simulink model "sampleModel1766"  (R2023a)
settings: Solver=VariableStepAuto  StartTime=0.0  StopTime=10.0  RelTol=1e-3
libraries: hdlsllib x6, simulink x2
settings Model: Creator=user1  LastModifiedBy=user1

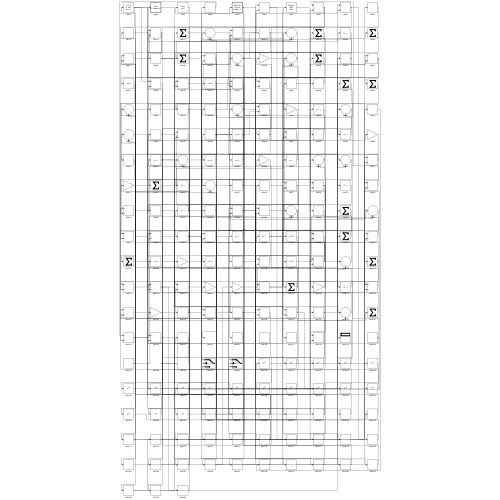
[thumbnail: Simulink's stored preview of the top-level diagram]
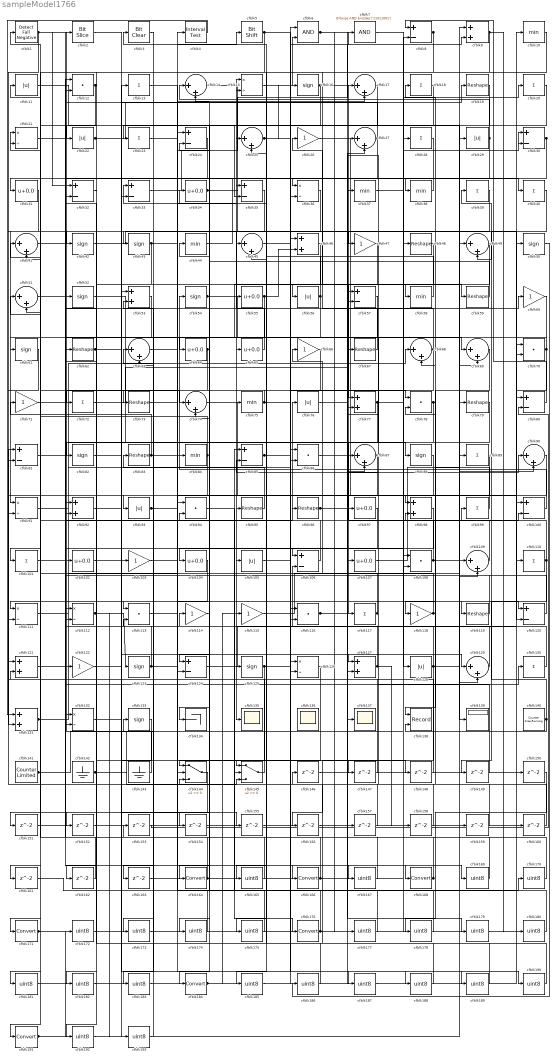
== system sampleModel1766 ==
  cfblk1 : hdlsllib/Logic and Bit Operations/Detect Fall Negative  vinit=0  OutDataTypeStr=boolean
  cfblk{10,37..38,44,58,75,84} (7 alike) : MinMax
  cfblk{8,24,30,32..33,35,57,80..81,85,100,106,120,124} (14 alike) : Sum  Inputs=+-
  cfblk{13,18,20,23,28,39..40,72,89,99,101,110,117,130} (14 alike) : Sum  Inputs=+
  cfblk{31,34,55,64..65,97,102,104,107} (9 alike) : Bias  Bias=0.0  SaturateOnIntegerOverflow=off
  cfblk{26,47,60,66,71,103,114..115,118,122} (10 alike) : Gain
  cfblk{11,22,29,56,76,93,105,128} (8 alike) : Abs  SaturateOnIntegerOverflow=off
  cfblk{12,70,78,86,94,108,113,116} (8 alike) : DotProduct  OutDataTypeStr=Inherit: Inherit via internal rule
  cfblk{14,17,25,27,41,45,49,51,63,68..69,74,87,90,109,129} (16 alike) : Sum  Inputs=|++
  cfblk{15,21,36,91,111..112,126,132} (8 alike) : Product  Inputs=*/  RndMeth=Zero  SaturateOnIntegerOverflow=on
  cfblk{19,48,59,62,67,73,79,83,95..96,119} (11 alike) : Reshape
  cfblk{9,46,53,77,92,98,121,127,131} (9 alike) : Sum
  cfblk{16,42..43,50,52,54,61,82,88,123,125,133} (12 alike) : Signum
  cfblk134 : Terminator
  cfblk135 : Scope
  cfblk136 : Scope
      settings: Floating=on
  cfblk137 : Scope
  cfblk138 : Record  FileSettingsInternal="{\"entries\":[{\"content\":{\"excelSettings\":{\"content\":{},\"type\":\"Streamout.ExcelSettings\"}},\"type\":\"Streamout.FileSettingStorage\",\"uuid\":\"\"}],\"packageUris\":[\"http:\\/\\/schema.mathworks.com\\/mf0\\/streamout_blocks\\/R2020a\"],\"version\":\"1.0\"}"  Layout=[1 1]  SignalsInternal="{\"entries\":[{\"content\":{\"signals\":[{\"content\":{\"blockPath\":[],\"dimensions\":[1],\"domain\":\"\",\"lineColor\":\"#a2142f\",\"plots\":[1],\"port\":1,\"signalID\":3847,\"signalName\":\"XY Graph:1\"},\"type\":\"RecordBlkView.Signal\",\"uuid\":\"\"},{\"content\":{\"blockPath\":[],\"dimensions\":[1],\"domain\":\"\",\"lineColor\":\"#139fff\",\"plots\":[1],\"port\":2,\"signalID\":3850,\"signalName\":\"XY Graph:2\"},\"type\":\"RecordBlkView.Signal\",\"uuid\":\"\"}]},\"type\":\"RecordBlkView.InputSignals\",\"uuid\":\"\"}],\"packageUris\":[\"http:\\/\\/schema.mathworks.com\\/mf0\\/streamout_blocks\\/R2020a\"],\"version\":\"1.0\"}"  VisualizationBindings="{\"xyplotplugin\":{\"info\":[{\"series\":[{\"bindingParametersList\":[{\"parameter\":\"X-Axis\",\"signalID\":3847,\"signalName\":\"XY Graph:1\"},{\"parameter\":\"Y-Axis\",\"signalID\":3850,\"signalName\":\"XY Graph:2\"}],\"seriesID\":23511}],\"subplotID\":1}]}}"  CompatibilityTag=XY  st=-1
  cfblk139 : Display
  cfblk140 : hdlsllib/Sources/Counter Free-Running  NumBits=16  tsamp=-1
  cfblk141 : hdlsllib/Sources/Counter Limited  uplimit=7  tsamp=-1
  cfblk142 : Ground
  cfblk143 : Ground
  cfblk144 : Switch  SaturateOnIntegerOverflow=off  InputSameDT=off
  cfblk145 : Switch  SaturateOnIntegerOverflow=off  InputSameDT=off
  cfblk{146..163} (18 alike) : Delay  SampleTime=1
  cfblk{164,166,168,171,176,184,191} (7 alike) : DataTypeConversion  SaturateOnIntegerOverflow=off  RndMeth=Floor
  cfblk{165,167,169..170,172..175,177..183,185..190,192..193} (23 alike) : DataTypeConversion  OutDataTypeStr=uint8  SaturateOnIntegerOverflow=off  RndMeth=Floor
  cfblk2 : hdlsllib/Logic and Bit Operations/Bit Slice  lidx=7  ridx=0
  cfblk3 : simulink/Logic and Bit Operations/Bit Clear  iBit=0
      settings: LibrarySourceBlock=|
      | hdlsllib/Logic and Bit
      | Operations/Bit Clear
  cfblk4 : hdlsllib/Logic and Bit Operations/Interval Test  IntervalClosedRight=on  uplimit=0.5  IntervalClosedLeft=on  lowlimit=-0.5  OutDataTypeStr=boolean
  cfblk5 : hdlsllib/Logic and Bit Operations/Bit Shift  mode=Shift Left Logical  N=0
  cfblk6 : Logic  AllPortsSameDT=off  OutDataTypeStr=boolean
  cfblk7 : simulink/Logic and Bit Operations/Bitwise Operator  logicop=AND  UseBitMask=on  BitMask=bin2dec('11011001')  BitMaskRealWorld=Stored Integer
      settings: LibrarySourceBlock=|
      | hdlsllib/Logic and Bit
      | Operations/Bitwise
      | Operator
  wires:
  cfblk131/1 -> cfblk68/1, cfblk130/1
  cfblk35/1 -> cfblk135/1
  cfblk31/1 -> cfblk91/1
  cfblk140/1 -> cfblk39/1, cfblk138/2
  cfblk44/1 -> cfblk36/1
  cfblk80/1 -> cfblk8/1
  cfblk95/1 -> cfblk83/1
  cfblk109/1 -> cfblk17/1
  cfblk89/1 -> cfblk184/1
  cfblk43/1 -> cfblk72/1, cfblk167/1
  cfblk58/1 -> cfblk33/1
  cfblk97/1 -> cfblk106/1
  cfblk6/1 -> cfblk87/2, cfblk177/1
  cfblk77/1 -> cfblk117/1, cfblk20/1
  cfblk100/1 -> cfblk54/1
  cfblk65/1 -> cfblk15/1
  cfblk2/1 -> cfblk33/2
  cfblk85/1 -> cfblk147/1, cfblk169/1
  cfblk16/1 -> cfblk59/1, cfblk35/2
  cfblk96/1 -> cfblk97/1, cfblk100/2
  cfblk81/1 -> cfblk88/1
  cfblk29/1 -> cfblk14/1, cfblk116/2
  cfblk52/1 -> cfblk126/1
  cfblk106/1 -> cfblk63/1
  cfblk57/1 -> cfblk95/1
  cfblk93/1 -> cfblk119/1, cfblk98/1
  cfblk4/1 -> cfblk131/1
  cfblk27/1 -> cfblk105/1, cfblk12/2
  cfblk143/1 -> cfblk2/1
  cfblk76/1 -> cfblk137/1
  cfblk117/1 -> cfblk66/1, cfblk41/2
  cfblk108/1 -> cfblk76/1, cfblk98/2, cfblk90/2, cfblk21/1
  cfblk53/1 -> cfblk191/1
  cfblk141/1 -> cfblk107/1, cfblk41/1
  cfblk56/1 -> cfblk3/1, cfblk144/2
  cfblk38/1 -> cfblk31/1
  cfblk5/1 -> cfblk78/1, cfblk152/1
  cfblk120/1 -> cfblk102/1
  cfblk74/1 -> cfblk139/1
  cfblk130/1 -> cfblk106/2
  cfblk66/1 -> cfblk134/1
  cfblk25/1 -> cfblk16/1, cfblk190/1
  cfblk39/1 -> cfblk42/1
  cfblk36/1 -> cfblk91/2
  cfblk79/1 -> cfblk82/1
  cfblk123/1 -> cfblk52/1, cfblk57/1
  cfblk103/1 -> cfblk84/1
  cfblk12/1 -> cfblk22/1, cfblk161/1
  cfblk125/1 -> cfblk127/1, cfblk174/1
  cfblk129/1 -> cfblk44/1
  cfblk15/1 -> cfblk6/2
  cfblk8/1 -> cfblk145/1, cfblk181/1
  cfblk119/1 -> cfblk63/2
  cfblk26/1 -> cfblk110/1
  cfblk67/1 -> cfblk26/1
  cfblk128/1 -> cfblk74/2, cfblk109/2, cfblk156/1
  cfblk145/1 -> cfblk121/2
  cfblk33/1 -> cfblk9/2
  cfblk41/1 -> cfblk74/1
  cfblk127/1 -> cfblk112/1, cfblk158/1
  cfblk75/1 -> cfblk120/1, cfblk73/1
  cfblk19/1 -> cfblk126/2
  cfblk7/1 -> cfblk128/1
  cfblk70/1 -> cfblk120/2, cfblk61/1
  cfblk113/1 -> cfblk17/2
  cfblk20/1 -> cfblk64/1
  cfblk54/1 -> cfblk69/1, cfblk58/1, cfblk69/2
  cfblk142/1 -> cfblk48/1, cfblk145/3
  cfblk49/1 -> cfblk77/1
  cfblk40/1 -> cfblk49/2
  cfblk83/1 -> cfblk11/1, cfblk25/1, cfblk21/2
  cfblk68/1 -> cfblk37/1, cfblk144/1
  cfblk90/1 -> cfblk124/1
  cfblk107/1 -> cfblk29/1
  cfblk14/1 -> cfblk80/1
  cfblk62/1 -> cfblk124/2, cfblk15/2
  cfblk99/1 -> cfblk68/2
  cfblk124/1 -> cfblk10/1
  cfblk42/1 -> cfblk47/1
  cfblk112/1 -> cfblk123/1, cfblk193/1
  cfblk61/1 -> cfblk81/2
  cfblk11/1 -> cfblk109/1
  cfblk64/1 -> cfblk14/2, cfblk101/1
  cfblk1/1 -> cfblk40/1, cfblk32/1, cfblk111/2, cfblk108/2
  cfblk28/1 -> cfblk171/1
  cfblk59/1 -> cfblk34/1
  cfblk69/1 -> cfblk138/1
  cfblk91/1 -> cfblk46/1
  cfblk21/1 -> cfblk38/1
  cfblk22/1 -> cfblk19/1, cfblk127/2, cfblk125/1
  cfblk55/1 -> cfblk93/1, cfblk25/2, cfblk46/2
  cfblk10/1 -> cfblk56/1
  cfblk63/1 -> cfblk35/1
  cfblk111/1 -> cfblk4/1
  cfblk118/1 -> cfblk18/1, cfblk32/2
  cfblk105/1 -> cfblk7/1
  cfblk92/1 -> cfblk168/1
  cfblk102/1 -> cfblk13/1
  cfblk17/1 -> cfblk55/1
  cfblk121/1 -> cfblk96/1
  cfblk116/1 -> cfblk67/1, cfblk90/1
  cfblk114/1 -> cfblk164/1
  cfblk87/1 -> cfblk131/2, cfblk85/2
  cfblk71/1 -> cfblk166/1
  cfblk9/1 -> cfblk163/1, cfblk180/1
  cfblk60/1 -> cfblk87/1
  cfblk104/1 -> cfblk111/1
  cfblk94/1 -> cfblk176/1
  cfblk78/1 -> cfblk118/1, cfblk113/1
  cfblk3/1 -> cfblk23/1
  cfblk30/1 -> cfblk36/2, cfblk75/1
  cfblk23/1 -> cfblk5/1
  cfblk110/1 -> cfblk99/1, cfblk149/1
  cfblk18/1 -> cfblk43/1
  cfblk73/1 -> cfblk129/1
  cfblk115/1 -> cfblk30/1
  cfblk37/1 -> cfblk30/2
  cfblk72/1 -> cfblk27/2
  cfblk51/1 -> cfblk65/1
  cfblk84/1 -> cfblk51/2, cfblk112/2
  cfblk34/1 -> cfblk79/1, cfblk104/1
  cfblk101/1 -> cfblk60/1
  cfblk146/1 -> cfblk70/2
  cfblk147/1 -> cfblk121/1
  cfblk132/1 -> cfblk148/1
  cfblk148/1 -> cfblk51/1
  cfblk149/1 -> cfblk77/2
  cfblk144/1 -> cfblk151/1
  cfblk151/1 -> cfblk9/1
  cfblk152/1 -> cfblk100/1
  cfblk153/1 -> cfblk80/2
  cfblk98/1 -> cfblk154/1
  cfblk154/1 -> cfblk6/1
  cfblk82/1 -> cfblk155/1
  cfblk155/1 -> cfblk8/2
  cfblk156/1 -> cfblk49/1
  cfblk157/1 -> cfblk12/1
  cfblk158/1 -> cfblk81/1
  cfblk159/1 -> cfblk27/1
  cfblk160/1 -> cfblk78/2
  cfblk32/1 -> cfblk162/1
  cfblk162/1 -> cfblk1/1
  cfblk163/1 -> cfblk145/2
  cfblk164/1 -> cfblk62/1, cfblk108/1
  cfblk47/1 -> cfblk165/1
  cfblk165/1 -> cfblk114/1
  cfblk166/1 -> cfblk153/1, cfblk113/2, cfblk132/2
  cfblk167/1 -> cfblk71/1
  cfblk168/1 -> cfblk116/1, cfblk132/1
  cfblk169/1 -> cfblk92/1
  cfblk161/1 -> cfblk170/1
  cfblk170/1 -> cfblk92/2
  cfblk171/1 -> cfblk160/1, cfblk159/1
  cfblk172/1 -> cfblk28/1
  cfblk24/1 -> cfblk173/1
  cfblk173/1 -> cfblk150/1
  cfblk174/1 -> cfblk24/1
  cfblk46/1 -> cfblk175/1
  cfblk175/1 -> cfblk24/2
  cfblk176/1 -> cfblk57/2, cfblk144/3, cfblk85/1
  cfblk177/1 -> cfblk94/1
  cfblk150/1 -> cfblk178/1
  cfblk178/1 -> cfblk94/2
  cfblk86/1 -> cfblk179/1
  cfblk179/1 -> cfblk70/1
  cfblk180/1 -> cfblk86/1
  cfblk181/1 -> cfblk86/2
  cfblk133/1 -> cfblk182/1
  cfblk182/1 -> cfblk103/1
  cfblk88/1 -> cfblk183/1
  cfblk183/1 -> cfblk133/1
  cfblk184/1 -> cfblk157/1, cfblk115/1
  cfblk126/1 -> cfblk185/1
  cfblk185/1 -> cfblk89/1
  cfblk50/1 -> cfblk186/1
  cfblk186/1 -> cfblk122/1
  cfblk13/1 -> cfblk187/1
  cfblk187/1 -> cfblk50/1
  cfblk45/1 -> cfblk188/1
  cfblk188/1 -> cfblk146/1
  cfblk122/1 -> cfblk189/1
  cfblk189/1 -> cfblk45/1
  cfblk190/1 -> cfblk45/2
  cfblk191/1 -> cfblk172/1, cfblk129/2
  cfblk48/1 -> cfblk192/1
  cfblk192/1 -> cfblk53/1
  cfblk193/1 -> cfblk53/2
